simulink model "fukt_test"  (R2023b)
settings: Solver=FixedStepAuto  StartTime=0.0  StopTime=inf  FixedStep=0.5  MaxStep=1  MinStep=1  RelTol=1e-3
undefined symbols (not defined in the file or in its folder): BOOL, DINT, OTL, slplc
libraries: arduinolib x3
(part 5 of 6)

== system fukt_test/PLC Controller Suite/__Logic/Fukt logic/Program/__Logic/OTU1/RungInOverride/ForceRungInFalseRead/__CoreLabelRead ==
  DataRead : DataStoreRead  DataStoreName=x_PLCLabel__s4_3653__Force_RungIn_False  IndexOptions=Index vector (dialog)  Indices=1  OutputSizes=1
  Out1 : Outport  VectorParamsAs1DForOutWhenUnconnected=off
  wires:
  DataRead/1 -> Out1/1

== system fukt_test/PLC Controller Suite/__Logic/Fukt logic/Program/__Logic/OTU2/Instruction_Enable/Rung-condition-in is true/__CoreVarWrite ==
  u : Inport
  DataWrite : DataStoreWrite  DataStoreName=xxx_PLC_VAR_fukt_bool  IndexOptions=Index vector (dialog)  Indices=1  OutputSizes=1
  wires:
  u/1 -> DataWrite/1

== system fukt_test/PLC Controller Suite/__Logic/Fukt logic/Program/__Logic/OTU2/RungInOverride/ForceRungInFalseRead/__CoreLabelRead ==
  DataRead : DataStoreRead  DataStoreName=x_PLCLabel__s4_3653__Force_RungIn_False  IndexOptions=Index vector (dialog)  Indices=1  OutputSizes=1
  Out1 : Outport  VectorParamsAs1DForOutWhenUnconnected=off
  wires:
  DataRead/1 -> Out1/1

== system fukt_test/PLC Controller Suite/__Logic/Fukt logic/Program/__Logic/TON/Instruction_Enable/Initialize Function/VarWrite ==
  In1 : Inport
  __CoreVarWrite : Subsystem  Tag=CoreVarWriteBlock  DisableCoverage=on  TreatAsAtomicUnit=on  mask{PLCBlockType=CoreVarWrite}
      mask init:
      | slplc.callbacks.initCoreVariable(gcb, 'write');
      mask Help: web([docroot '/plccoder/ref/__corevarwrite' '.html']);
      mask DialogControl PLCBlockTitle Prompt: Core Variable Write
  wires:
  In1/1 -> __CoreVarWrite/1(u)

== system fukt_test/PLC Controller Suite/__Logic/Fukt logic/Program/__Logic/TON/Instruction_Enable/Initialize Function/VarWrite1 ==
  In1 : Inport
  __CoreVarWrite : Subsystem  Tag=CoreVarWriteBlock  DisableCoverage=on  TreatAsAtomicUnit=on  mask{PLCBlockType=CoreVarWrite}
      mask init:
      | slplc.callbacks.initCoreVariable(gcb, 'write');
      mask Help: web([docroot '/plccoder/ref/__corevarwrite' '.html']);
      mask DialogControl PLCBlockTitle Prompt: Core Variable Write
  wires:
  In1/1 -> __CoreVarWrite/1(u)

== system fukt_test/PLC Controller Suite/__Logic/Fukt logic/Program/__Logic/TON/Instruction_Enable/Initialize Function/VarWrite2 ==
  In1 : Inport
  __CoreVarWrite : Subsystem  Tag=CoreVarWriteBlock  DisableCoverage=on  TreatAsAtomicUnit=on  mask{PLCBlockType=CoreVarWrite}
      mask init:
      | slplc.callbacks.initCoreVariable(gcb, 'write');
      mask Help: web([docroot '/plccoder/ref/__corevarwrite' '.html']);
      mask DialogControl PLCBlockTitle Prompt: Core Variable Write
  wires:
  In1/1 -> __CoreVarWrite/1(u)

== system fukt_test/PLC Controller Suite/__Logic/Fukt logic/Program/__Logic/TON/Instruction_Enable/Initialize Function/VarWrite3 ==
  In1 : Inport
  __CoreVarWrite : Subsystem  Tag=CoreVarWriteBlock  DisableCoverage=on  TreatAsAtomicUnit=on  mask{PLCBlockType=CoreVarWrite}
      mask init:
      | slplc.callbacks.initCoreVariable(gcb, 'write');
      mask Help: web([docroot '/plccoder/ref/__corevarwrite' '.html']);
      mask DialogControl PLCBlockTitle Prompt: Core Variable Write
  wires:
  In1/1 -> __CoreVarWrite/1(u)

== system fukt_test/PLC Controller Suite/__Logic/Fukt logic/Program/__Logic/TON/RungInOverride/ForceRungInFalseRead/__CoreLabelRead ==
  DataRead : DataStoreRead  DataStoreName=x_PLCLabel__s4_3653__Force_RungIn_False  IndexOptions=Index vector (dialog)  Indices=1  OutputSizes=1
  Out1 : Outport  VectorParamsAs1DForOutWhenUnconnected=off
  wires:
  DataRead/1 -> Out1/1

== system fukt_test/PLC Controller Suite/__Logic/Fukt logic/Program/__Logic/XIC1/RungInOverride/ForceRungInFalseRead/__CoreLabelRead ==
  DataRead : DataStoreRead  DataStoreName=x_PLCLabel__s4_3653__Force_RungIn_False  IndexOptions=Index vector (dialog)  Indices=1  OutputSizes=1
  Out1 : Outport  VectorParamsAs1DForOutWhenUnconnected=off
  wires:
  DataRead/1 -> Out1/1

== system fukt_test/PLC Controller Suite/__Logic/Fukt logic/Program/__Logic/XIC2/RungInOverride/ForceRungInFalseRead/__CoreLabelRead ==
  DataRead : DataStoreRead  DataStoreName=x_PLCLabel__s4_3653__Force_RungIn_False  IndexOptions=Index vector (dialog)  Indices=1  OutputSizes=1
  Out1 : Outport  VectorParamsAs1DForOutWhenUnconnected=off
  wires:
  DataRead/1 -> Out1/1

== system fukt_test/PLC Controller Suite/__Logic/Fukt logic/Program/__Logic/XIC3/RungInOverride/ForceRungInFalseRead/__CoreLabelRead ==
  DataRead : DataStoreRead  DataStoreName=x_PLCLabel__s4_3653__Force_RungIn_False  IndexOptions=Index vector (dialog)  Indices=1  OutputSizes=1
  Out1 : Outport  VectorParamsAs1DForOutWhenUnconnected=off
  wires:
  DataRead/1 -> Out1/1

== system fukt_test/PLC Controller Suite/__Logic/Fukt sampling/Fuktmätare sampling/__Logic/MOV/RungInOverride/ForceRungInFalseRead/__CoreLabelRead ==
  DataRead : DataStoreRead  DataStoreName=x_PLCLabel__s4_3653__Force_RungIn_False  IndexOptions=Index vector (dialog)  Indices=1  OutputSizes=1
  Out1 : Outport  VectorParamsAs1DForOutWhenUnconnected=off
  wires:
  DataRead/1 -> Out1/1

== system fukt_test/PLC Controller Suite/__Logic/Fukt sampling/Fuktmätare sampling/__Logic/MOV/RungOutOverride/BlockEnableRead/__CoreLabelRead ==
  DataRead : DataStoreRead  DataStoreName=x_PLCLabel__s4_3653__Block_Enable  IndexOptions=Index vector (dialog)  Indices=1  OutputSizes=1
  Out1 : Outport  VectorParamsAs1DForOutWhenUnconnected=off
  wires:
  DataRead/1 -> Out1/1

== system fukt_test/PLC Controller Suite/__Logic/Fukt sampling/Fuktmätare sampling/__Logic/MOV/RungOutOverride/VariableWriteEnableWrite/__CoreLabelWrite ==
  In1 : Inport
  DataWrite : DataStoreWrite  DataStoreName=x_PLCLabel__s4_3653__Variable_Write_Enable  IndexOptions=Index vector (dialog)  Indices=1  OutputSizes=1
  wires:
  In1/1 -> DataWrite/1

== system fukt_test/PLC Controller Suite/__Logic/Fukt sampling/Fuktmätare sampling/__Logic/OTL/Instruction_Enable/Rung-condition-in is true/__CoreVarWrite ==
  u : Inport
  DataWrite : DataStoreWrite  DataStoreName=xxx_PLC_VAR_fukt_polling  IndexOptions=Index vector (dialog)  Indices=1  OutputSizes=1
  wires:
  u/1 -> DataWrite/1

== system fukt_test/PLC Controller Suite/__Logic/Fukt sampling/Fuktmätare sampling/__Logic/OTL/RungInOverride/ForceRungInFalseRead/__CoreLabelRead ==
  DataRead : DataStoreRead  DataStoreName=x_PLCLabel__s4_3653__Force_RungIn_False  IndexOptions=Index vector (dialog)  Indices=1  OutputSizes=1
  Out1 : Outport  VectorParamsAs1DForOutWhenUnconnected=off
  wires:
  DataRead/1 -> Out1/1

== system fukt_test/PLC Controller Suite/__Logic/Fukt sampling/Fuktmätare sampling/__Logic/OTL1/Instruction_Enable/Rung-condition-in is true/__CoreVarWrite ==
  u : Inport
  DataWrite : DataStoreWrite  DataStoreName=xxx_PLC_VAR_fukt_power  IndexOptions=Index vector (dialog)  Indices=1  OutputSizes=1
  wires:
  u/1 -> DataWrite/1

== system fukt_test/PLC Controller Suite/__Logic/Fukt sampling/Fuktmätare sampling/__Logic/OTL1/RungInOverride/ForceRungInFalseRead/__CoreLabelRead ==
  DataRead : DataStoreRead  DataStoreName=x_PLCLabel__s4_3653__Force_RungIn_False  IndexOptions=Index vector (dialog)  Indices=1  OutputSizes=1
  Out1 : Outport  VectorParamsAs1DForOutWhenUnconnected=off
  wires:
  DataRead/1 -> Out1/1

== system fukt_test/PLC Controller Suite/__Logic/Fukt sampling/Fuktmätare sampling/__Logic/OTU/Instruction_Enable/Rung-condition-in is true/__CoreVarWrite ==
  u : Inport
  DataWrite : DataStoreWrite  DataStoreName=xxx_PLC_VAR_fukt_power  IndexOptions=Index vector (dialog)  Indices=1  OutputSizes=1
  wires:
  u/1 -> DataWrite/1

== system fukt_test/PLC Controller Suite/__Logic/Fukt sampling/Fuktmätare sampling/__Logic/OTU/RungInOverride/ForceRungInFalseRead/__CoreLabelRead ==
  DataRead : DataStoreRead  DataStoreName=x_PLCLabel__s4_3653__Force_RungIn_False  IndexOptions=Index vector (dialog)  Indices=1  OutputSizes=1
  Out1 : Outport  VectorParamsAs1DForOutWhenUnconnected=off
  wires:
  DataRead/1 -> Out1/1

== system fukt_test/PLC Controller Suite/__Logic/Fukt sampling/Fuktmätare sampling/__Logic/RES/Instruction_Enable/Rung-condition-in is true/__CoreVarRead ==
  DataRead : DataStoreRead  DataStoreName=xxx_PLC_VAR_Fukt_periodicity  IndexOptions=Index vector (dialog)  Indices=1  OutputSizes=1
  y : Outport  VectorParamsAs1DForOutWhenUnconnected=off
  wires:
  DataRead/1 -> y/1

== system fukt_test/PLC Controller Suite/__Logic/Fukt sampling/Fuktmätare sampling/__Logic/RES/Instruction_Enable/Rung-condition-in is true/__CoreVarWrite ==
  u : Inport
  DataWrite : DataStoreWrite  DataStoreName=xxx_PLC_VAR_Fukt_periodicity  IndexOptions=Index vector (dialog)  Indices=1  OutputSizes=1
  wires:
  u/1 -> DataWrite/1

== system fukt_test/PLC Controller Suite/__Logic/Fukt sampling/Fuktmätare sampling/__Logic/RES/RungInOverride/ForceRungInFalseRead/__CoreLabelRead ==
  DataRead : DataStoreRead  DataStoreName=x_PLCLabel__s4_3653__Force_RungIn_False  IndexOptions=Index vector (dialog)  Indices=1  OutputSizes=1
  Out1 : Outport  VectorParamsAs1DForOutWhenUnconnected=off
  wires:
  DataRead/1 -> Out1/1

== system fukt_test/PLC Controller Suite/__Logic/Fukt sampling/Fuktmätare sampling/__Logic/TON/Instruction_Enable/Initialize Function/VarWrite ==
  In1 : Inport
  __CoreVarWrite : Subsystem  Tag=CoreVarWriteBlock  DisableCoverage=on  TreatAsAtomicUnit=on  mask{PLCBlockType=CoreVarWrite}
      mask init:
      | slplc.callbacks.initCoreVariable(gcb, 'write');
      mask Help: web([docroot '/plccoder/ref/__corevarwrite' '.html']);
      mask DialogControl PLCBlockTitle Prompt: Core Variable Write
  wires:
  In1/1 -> __CoreVarWrite/1(u)

== system fukt_test/PLC Controller Suite/__Logic/Fukt sampling/Fuktmätare sampling/__Logic/TON/Instruction_Enable/Initialize Function/VarWrite1 ==
  In1 : Inport
  __CoreVarWrite : Subsystem  Tag=CoreVarWriteBlock  DisableCoverage=on  TreatAsAtomicUnit=on  mask{PLCBlockType=CoreVarWrite}
      mask init:
      | slplc.callbacks.initCoreVariable(gcb, 'write');
      mask Help: web([docroot '/plccoder/ref/__corevarwrite' '.html']);
      mask DialogControl PLCBlockTitle Prompt: Core Variable Write
  wires:
  In1/1 -> __CoreVarWrite/1(u)

== system fukt_test/PLC Controller Suite/__Logic/Fukt sampling/Fuktmätare sampling/__Logic/TON/Instruction_Enable/Initialize Function/VarWrite2 ==
  In1 : Inport
  __CoreVarWrite : Subsystem  Tag=CoreVarWriteBlock  DisableCoverage=on  TreatAsAtomicUnit=on  mask{PLCBlockType=CoreVarWrite}
      mask init:
      | slplc.callbacks.initCoreVariable(gcb, 'write');
      mask Help: web([docroot '/plccoder/ref/__corevarwrite' '.html']);
      mask DialogControl PLCBlockTitle Prompt: Core Variable Write
  wires:
  In1/1 -> __CoreVarWrite/1(u)

== system fukt_test/PLC Controller Suite/__Logic/Fukt sampling/Fuktmätare sampling/__Logic/TON/Instruction_Enable/Initialize Function/VarWrite3 ==
  In1 : Inport
  __CoreVarWrite : Subsystem  Tag=CoreVarWriteBlock  DisableCoverage=on  TreatAsAtomicUnit=on  mask{PLCBlockType=CoreVarWrite}
      mask init:
      | slplc.callbacks.initCoreVariable(gcb, 'write');
      mask Help: web([docroot '/plccoder/ref/__corevarwrite' '.html']);
      mask DialogControl PLCBlockTitle Prompt: Core Variable Write
  wires:
  In1/1 -> __CoreVarWrite/1(u)

== system fukt_test/PLC Controller Suite/__Logic/Fukt sampling/Fuktmätare sampling/__Logic/TON/RungInOverride/ForceRungInFalseRead/__CoreLabelRead ==
  DataRead : DataStoreRead  DataStoreName=x_PLCLabel__s4_3653__Force_RungIn_False  IndexOptions=Index vector (dialog)  Indices=1  OutputSizes=1
  Out1 : Outport  VectorParamsAs1DForOutWhenUnconnected=off
  wires:
  DataRead/1 -> Out1/1

== system fukt_test/PLC Controller Suite/__Logic/Fukt sampling/Fuktmätare sampling/__Logic/TON1/Instruction_Enable/Initialize Function/VarWrite ==
  In1 : Inport
  __CoreVarWrite : Subsystem  Tag=CoreVarWriteBlock  DisableCoverage=on  TreatAsAtomicUnit=on  mask{PLCBlockType=CoreVarWrite}
      mask init:
      | slplc.callbacks.initCoreVariable(gcb, 'write');
      mask Help: web([docroot '/plccoder/ref/__corevarwrite' '.html']);
      mask DialogControl PLCBlockTitle Prompt: Core Variable Write
  wires:
  In1/1 -> __CoreVarWrite/1(u)

== system fukt_test/PLC Controller Suite/__Logic/Fukt sampling/Fuktmätare sampling/__Logic/TON1/Instruction_Enable/Initialize Function/VarWrite1 ==
  In1 : Inport
  __CoreVarWrite : Subsystem  Tag=CoreVarWriteBlock  DisableCoverage=on  TreatAsAtomicUnit=on  mask{PLCBlockType=CoreVarWrite}
      mask init:
      | slplc.callbacks.initCoreVariable(gcb, 'write');
      mask Help: web([docroot '/plccoder/ref/__corevarwrite' '.html']);
      mask DialogControl PLCBlockTitle Prompt: Core Variable Write
  wires:
  In1/1 -> __CoreVarWrite/1(u)

== system fukt_test/PLC Controller Suite/__Logic/Fukt sampling/Fuktmätare sampling/__Logic/TON1/Instruction_Enable/Initialize Function/VarWrite2 ==
  In1 : Inport
  __CoreVarWrite : Subsystem  Tag=CoreVarWriteBlock  DisableCoverage=on  TreatAsAtomicUnit=on  mask{PLCBlockType=CoreVarWrite}
      mask init:
      | slplc.callbacks.initCoreVariable(gcb, 'write');
      mask Help: web([docroot '/plccoder/ref/__corevarwrite' '.html']);
      mask DialogControl PLCBlockTitle Prompt: Core Variable Write
  wires:
  In1/1 -> __CoreVarWrite/1(u)

== system fukt_test/PLC Controller Suite/__Logic/Fukt sampling/Fuktmätare sampling/__Logic/TON1/Instruction_Enable/Initialize Function/VarWrite3 ==
  In1 : Inport
  __CoreVarWrite : Subsystem  Tag=CoreVarWriteBlock  DisableCoverage=on  TreatAsAtomicUnit=on  mask{PLCBlockType=CoreVarWrite}
      mask init:
      | slplc.callbacks.initCoreVariable(gcb, 'write');
      mask Help: web([docroot '/plccoder/ref/__corevarwrite' '.html']);
      mask DialogControl PLCBlockTitle Prompt: Core Variable Write
  wires:
  In1/1 -> __CoreVarWrite/1(u)

== system fukt_test/PLC Controller Suite/__Logic/Fukt sampling/Fuktmätare sampling/__Logic/TON1/RungInOverride/ForceRungInFalseRead/__CoreLabelRead ==
  DataRead : DataStoreRead  DataStoreName=x_PLCLabel__s4_3653__Force_RungIn_False  IndexOptions=Index vector (dialog)  Indices=1  OutputSizes=1
  Out1 : Outport  VectorParamsAs1DForOutWhenUnconnected=off
  wires:
  DataRead/1 -> Out1/1

== system fukt_test/PLC Controller Suite/__Logic/Fukt sampling/Fuktmätare sampling/__Logic/XIC1/RungInOverride/ForceRungInFalseRead/__CoreLabelRead ==
  DataRead : DataStoreRead  DataStoreName=x_PLCLabel__s4_3653__Force_RungIn_False  IndexOptions=Index vector (dialog)  Indices=1  OutputSizes=1
  Out1 : Outport  VectorParamsAs1DForOutWhenUnconnected=off
  wires:
  DataRead/1 -> Out1/1

== system fukt_test/PLC Controller Suite/__Logic/Fukt sampling/Fuktmätare sampling/__Logic/XIC2/RungInOverride/ForceRungInFalseRead/__CoreLabelRead ==
  DataRead : DataStoreRead  DataStoreName=x_PLCLabel__s4_3653__Force_RungIn_False  IndexOptions=Index vector (dialog)  Indices=1  OutputSizes=1
  Out1 : Outport  VectorParamsAs1DForOutWhenUnconnected=off
  wires:
  DataRead/1 -> Out1/1

== system fukt_test/PLC Controller Suite/__Logic/Fukt logic/Program/__Logic/TON/Instruction_Enable/Initialize Function/VarWrite/__CoreVarWrite ==
  u : Inport
  DataWrite : DataStoreWrite  DataStoreName=xxx_PLC_VAR_orange_led_timer_1  DataStoreElements=xxx_PLC_VAR_orange_led_timer_1.ACC  IndexOptions=Index vector (dialog)  Indices=1  OutputSizes=1
  wires:
  u/1 -> DataWrite/1

== system fukt_test/PLC Controller Suite/__Logic/Fukt logic/Program/__Logic/TON/Instruction_Enable/Initialize Function/VarWrite1/__CoreVarWrite ==
  u : Inport
  DataWrite : DataStoreWrite  DataStoreName=xxx_PLC_VAR_orange_led_timer_1  DataStoreElements=xxx_PLC_VAR_orange_led_timer_1.EN  IndexOptions=Index vector (dialog)  Indices=1  OutputSizes=1
  wires:
  u/1 -> DataWrite/1

== system fukt_test/PLC Controller Suite/__Logic/Fukt logic/Program/__Logic/TON/Instruction_Enable/Initialize Function/VarWrite2/__CoreVarWrite ==
  u : Inport
  DataWrite : DataStoreWrite  DataStoreName=xxx_PLC_VAR_orange_led_timer_1  DataStoreElements=xxx_PLC_VAR_orange_led_timer_1.TT  IndexOptions=Index vector (dialog)  Indices=1  OutputSizes=1
  wires:
  u/1 -> DataWrite/1

== system fukt_test/PLC Controller Suite/__Logic/Fukt logic/Program/__Logic/TON/Instruction_Enable/Initialize Function/VarWrite3/__CoreVarWrite ==
  u : Inport
  DataWrite : DataStoreWrite  DataStoreName=xxx_PLC_VAR_orange_led_timer_1  DataStoreElements=xxx_PLC_VAR_orange_led_timer_1.DN  IndexOptions=Index vector (dialog)  Indices=1  OutputSizes=1
  wires:
  u/1 -> DataWrite/1

== system fukt_test/PLC Controller Suite/__Logic/Fukt sampling/Fuktmätare sampling/__Logic/TON/Instruction_Enable/Initialize Function/VarWrite/__CoreVarWrite ==
  u : Inport
  DataWrite : DataStoreWrite  DataStoreName=xxx_PLC_VAR_Fukt_periodicity  DataStoreElements=xxx_PLC_VAR_Fukt_periodicity.ACC  IndexOptions=Index vector (dialog)  Indices=1  OutputSizes=1
  wires:
  u/1 -> DataWrite/1

== system fukt_test/PLC Controller Suite/__Logic/Fukt sampling/Fuktmätare sampling/__Logic/TON/Instruction_Enable/Initialize Function/VarWrite1/__CoreVarWrite ==
  u : Inport
  DataWrite : DataStoreWrite  DataStoreName=xxx_PLC_VAR_Fukt_periodicity  DataStoreElements=xxx_PLC_VAR_Fukt_periodicity.EN  IndexOptions=Index vector (dialog)  Indices=1  OutputSizes=1
  wires:
  u/1 -> DataWrite/1

== system fukt_test/PLC Controller Suite/__Logic/Fukt sampling/Fuktmätare sampling/__Logic/TON/Instruction_Enable/Initialize Function/VarWrite2/__CoreVarWrite ==
  u : Inport
  DataWrite : DataStoreWrite  DataStoreName=xxx_PLC_VAR_Fukt_periodicity  DataStoreElements=xxx_PLC_VAR_Fukt_periodicity.TT  IndexOptions=Index vector (dialog)  Indices=1  OutputSizes=1
  wires:
  u/1 -> DataWrite/1

== system fukt_test/PLC Controller Suite/__Logic/Fukt sampling/Fuktmätare sampling/__Logic/TON/Instruction_Enable/Initialize Function/VarWrite3/__CoreVarWrite ==
  u : Inport
  DataWrite : DataStoreWrite  DataStoreName=xxx_PLC_VAR_Fukt_periodicity  DataStoreElements=xxx_PLC_VAR_Fukt_periodicity.DN  IndexOptions=Index vector (dialog)  Indices=1  OutputSizes=1
  wires:
  u/1 -> DataWrite/1

== system fukt_test/PLC Controller Suite/__Logic/Fukt sampling/Fuktmätare sampling/__Logic/TON1/Instruction_Enable/Initialize Function/VarWrite/__CoreVarWrite ==
  u : Inport
  DataWrite : DataStoreWrite  DataStoreName=xxx_PLC_VAR_d13_wait  DataStoreElements=xxx_PLC_VAR_d13_wait.ACC  IndexOptions=Index vector (dialog)  Indices=1  OutputSizes=1
  wires:
  u/1 -> DataWrite/1

== system fukt_test/PLC Controller Suite/__Logic/Fukt sampling/Fuktmätare sampling/__Logic/TON1/Instruction_Enable/Initialize Function/VarWrite1/__CoreVarWrite ==
  u : Inport
  DataWrite : DataStoreWrite  DataStoreName=xxx_PLC_VAR_d13_wait  DataStoreElements=xxx_PLC_VAR_d13_wait.EN  IndexOptions=Index vector (dialog)  Indices=1  OutputSizes=1
  wires:
  u/1 -> DataWrite/1

== system fukt_test/PLC Controller Suite/__Logic/Fukt sampling/Fuktmätare sampling/__Logic/TON1/Instruction_Enable/Initialize Function/VarWrite2/__CoreVarWrite ==
  u : Inport
  DataWrite : DataStoreWrite  DataStoreName=xxx_PLC_VAR_d13_wait  DataStoreElements=xxx_PLC_VAR_d13_wait.TT  IndexOptions=Index vector (dialog)  Indices=1  OutputSizes=1
  wires:
  u/1 -> DataWrite/1

== system fukt_test/PLC Controller Suite/__Logic/Fukt sampling/Fuktmätare sampling/__Logic/TON1/Instruction_Enable/Initialize Function/VarWrite3/__CoreVarWrite ==
  u : Inport
  DataWrite : DataStoreWrite  DataStoreName=xxx_PLC_VAR_d13_wait  DataStoreElements=xxx_PLC_VAR_d13_wait.DN  IndexOptions=Index vector (dialog)  Indices=1  OutputSizes=1
  wires:
  u/1 -> DataWrite/1

== matlab function fukt_test/PLC Controller Suite/__Logic/Fukt sampling/Fuktmätare sampling/__Logic/Power Rail Start/__Format ==
  data: RungOut input
function setBlockFormat(RungOut)
% set parent block colors
coder.extrinsic('slplc.utils.setBlockAppearance');
persistent isInit lastRungOut lastAnimation lastRungOutShow;

if isempty(isInit)
    isInit = true;
else
    isInit = false;
end

if isempty(lastRungOut)
    lastRungOut = RungOut;
end

if isempty(lastAnimation)
    lastAnimation = false;
end

if isempty(lastRungOutShow)
    lastRungOutShow = false;
end

[animation, dataShow] = slplc.utils.setBlockAppearance('set', '', {'black', 'black'}, {}, ...
    '', {'ForegroundColor', 'BackgroundColor'}, ...
    isInit,  ...
    true,  true, ...
    RungOut,   lastRungOut, ...
    RungOut,   lastRungOut, ...
    [],    [], ...
    lastAnimation, lastRungOutShow);

lastRungOut         = RungOut;
lastAnimation       = animation;
lastRungOutShow     = dataShow;
end

== matlab function fukt_test/PLC Controller Suite/__Logic/Fukt logic/Program/__Logic/TON/Instruction_Enable/__Logic ==
  data: EN output; TT output; RungIn input; PRE input; EN input; DN input; DN output; ACC output; ACC input; currentTime input; lastTime input
function [EN, TT, DN, ACC]  = TON(RungIn, PRE, EN, DN, ACC, currentTime, lastTime)
% TON algorithm

if RungIn
    % Rung-condition-in is True
    if PRE < 0 || ACC < 0
        error('slplc:TONError', '.PRE or .ACC cannot be negtive values');
    end
    TT = true;
    if ~DN
        if EN
            deltaT = currentTime - lastTime;
            ACC = ACC + cast(deltaT, class(ACC));
            if ACC == intmax(class(ACC)) || ACC >= PRE
                TT = false;
                DN = true;
            end
        end
    else
        TT = false;
    end
    EN = true;
    % True end
else
    % Rung-condition-in is False
    EN    = false;
    TT    = false;
    DN    = false;
    ACC   = cast(0, class(ACC));
    % False end
end

end

== matlab function fukt_test/PLC Controller Suite/__Logic/Fukt sampling/Fuktmätare sampling/__Logic/TON/Instruction_Enable/__Logic ==
  data: EN output; TT output; RungIn input; PRE input; EN input; DN input; DN output; ACC output; ACC input; currentTime input; lastTime input
function [EN, TT, DN, ACC]  = TON(RungIn, PRE, EN, DN, ACC, currentTime, lastTime)
% TON algorithm

if RungIn
    % Rung-condition-in is True
    if PRE < 0 || ACC < 0
        error('slplc:TONError', '.PRE or .ACC cannot be negtive values');
    end
    TT = true;
    if ~DN
        if EN
            deltaT = currentTime - lastTime;
            ACC = ACC + cast(deltaT, class(ACC));
            if ACC == intmax(class(ACC)) || ACC >= PRE
                TT = false;
                DN = true;
            end
        end
    else
        TT = false;
    end
    EN = true;
    % True end
else
    % Rung-condition-in is False
    EN    = false;
    TT    = false;
    DN    = false;
    ACC   = cast(0, class(ACC));
    % False end
end

end

== matlab function fukt_test/PLC Controller Suite/__Logic/Fukt sampling/Fuktmätare sampling/__Logic/TON/__Format ==
  data: BlockEnable input; RungIn input; RungOut input; data input
function setBlockFormat(BlockEnable, RungIn, RungOut, data)
% set parent block colors
coder.extrinsic('slplc.utils.setBlockAppearance');
persistent lastBlockEnable lastRungIn lastRungOut lastData isInit lastAnimation lastDataShow;
if isempty(lastBlockEnable)
    lastBlockEnable = true;
end
if isempty(lastRungIn)
    lastRungIn = false;
end
if isempty(lastRungOut)
    lastRungOut = false;
end
if isempty(lastData)
    lastData = data;
end
if isempty(isInit)
    isInit = true;
else
    isInit = false;
end
if isempty(lastAnimation)
    lastAnimation = false;
end
if isempty(lastDataShow)
    lastDataShow = false;
end

[animation, dataShow] = slplc.utils.setBlockAppearance('set', '%<PLCBlockType>: %<PLCOperandTag>', {}, {}, ...
    ' = ', {'ForegroundColor'}, ...
    isInit,  ...
    BlockEnable, lastBlockEnable, ...
    RungIn,  lastRungIn, ...
    RungOut, lastRungOut, ...
    data, lastData, ...
    lastAnimation, lastDataShow);

lastBlockEnable = BlockEnable;
lastRungIn      = RungIn;
lastRungOut     = RungOut;
lastData        = data;
lastAnimation   = animation;
lastDataShow    = dataShow;
end

== matlab function fukt_test/PLC Controller Suite/__Logic/Fukt sampling/Fuktmätare sampling/__Logic/Variable Read/__Format ==
  data: data input
function setBlockFormat(data)
% set parent block colors
coder.extrinsic('slplc.utils.setBlockAppearance');
persistent isInit lastData  lastAnimation lastDataShow;

if isempty(isInit)
    isInit = true;
else
    isInit = false;
end

if isempty(lastData)
    lastData = data;
end

if isempty(lastAnimation)
    lastAnimation = false;
end

if isempty(lastDataShow)
    lastDataShow = false;
end

[animation, dataShow] = slplc.utils.setBlockAppearance('set', '', {}, {}, ...
    '%<PLCOperandTag> = ', {}, ...
    isInit,  ...
    true,  true, ...
    false, false, ...
    false, false, ...
    data,  lastData, ...
    lastAnimation, lastDataShow);

lastData        = data;
lastAnimation   = animation;
lastDataShow    = dataShow;
end

== matlab function fukt_test/PLC Controller Suite/__Logic/Fukt logic/Program/__Logic/TON/__Format ==
  data: BlockEnable input; RungIn input; RungOut input; data input
function setBlockFormat(BlockEnable, RungIn, RungOut, data)
% set parent block colors
coder.extrinsic('slplc.utils.setBlockAppearance');
persistent lastBlockEnable lastRungIn lastRungOut lastData isInit lastAnimation lastDataShow;
if isempty(lastBlockEnable)
    lastBlockEnable = true;
end
if isempty(lastRungIn)
    lastRungIn = false;
end
if isempty(lastRungOut)
    lastRungOut = false;
end
if isempty(lastData)
    lastData = data;
end
if isempty(isInit)
    isInit = true;
else
    isInit = false;
end
if isempty(lastAnimation)
    lastAnimation = false;
end
if isempty(lastDataShow)
    lastDataShow = false;
end

[animation, dataShow] = slplc.utils.setBlockAppearance('set', '%<PLCBlockType>: %<PLCOperandTag>', {}, {}, ...
    ' = ', {'ForegroundColor'}, ...
    isInit,  ...
    BlockEnable, lastBlockEnable, ...
    RungIn,  lastRungIn, ...
    RungOut, lastRungOut, ...
    data, lastData, ...
    lastAnimation, lastDataShow);

lastBlockEnable = BlockEnable;
lastRungIn      = RungIn;
lastRungOut     = RungOut;
lastData        = data;
lastAnimation   = animation;
lastDataShow    = dataShow;
end

== matlab function fukt_test/PLC Controller Suite/__Logic/Fukt logic/Program/__Logic/OTU/__Format ==
  data: BlockEnable input; RungIn input; RungOut input; data input
function setBlockFormat(BlockEnable, RungIn, RungOut, data)

if data~=0 && data~=1
    error('slplc:inivalidBooleanValue', 'Invalid boolean value %d', data);
end
data = logical(data);

% set parent block colors
coder.extrinsic('slplc.utils.setBlockAppearance');
persistent lastBlockEnable lastRungIn lastRungOut lastData isInit lastAnimation lastDataShow;
if isempty(lastBlockEnable)
    lastBlockEnable = true;
end
if isempty(lastRungIn)
    lastRungIn = false;
end
if isempty(lastRungOut)
    lastRungOut = false;
end
if isempty(lastData)
    lastData = data;
end
if isempty(isInit)
    isInit = true;
else
    isInit = false;
end
if isempty(lastAnimation)
    lastAnimation = false;
end
if isempty(lastDataShow)
    lastDataShow = false;
end

[animation, dataShow] = slplc.utils.setBlockAppearance('set', '%<PLCOperandTag>', {}, {}, ...
    ' = ', {'ForegroundColor'}, ...
    isInit,  ...
    BlockEnable, lastBlockEnable, ...
    RungIn,  lastRungIn, ...
    RungOut, lastRungOut, ...
    data, lastData, ...
    lastAnimation, lastDataShow);

lastBlockEnable = BlockEnable;
lastRungIn      = RungIn;
lastRungOut     = RungOut;
lastData        = data;
lastAnimation   = animation;
lastDataShow    = dataShow;
end

== matlab function fukt_test/PLC Controller Suite/__Logic/Fukt logic/Program/__Logic/OTU1/__Format ==
  data: BlockEnable input; RungIn input; RungOut input; data input
function setBlockFormat(BlockEnable, RungIn, RungOut, data)

if data~=0 && data~=1
    error('slplc:inivalidBooleanValue', 'Invalid boolean value %d', data);
end
data = logical(data);

% set parent block colors
coder.extrinsic('slplc.utils.setBlockAppearance');
persistent lastBlockEnable lastRungIn lastRungOut lastData isInit lastAnimation lastDataShow;
if isempty(lastBlockEnable)
    lastBlockEnable = true;
end
if isempty(lastRungIn)
    lastRungIn = false;
end
if isempty(lastRungOut)
    lastRungOut = false;
end
if isempty(lastData)
    lastData = data;
end
if isempty(isInit)
    isInit = true;
else
    isInit = false;
end
if isempty(lastAnimation)
    lastAnimation = false;
end
if isempty(lastDataShow)
    lastDataShow = false;
end

[animation, dataShow] = slplc.utils.setBlockAppearance('set', '%<PLCOperandTag>', {}, {}, ...
    ' = ', {'ForegroundColor'}, ...
    isInit,  ...
    BlockEnable, lastBlockEnable, ...
    RungIn,  lastRungIn, ...
    RungOut, lastRungOut, ...
    data, lastData, ...
    lastAnimation, lastDataShow);

lastBlockEnable = BlockEnable;
lastRungIn      = RungIn;
lastRungOut     = RungOut;
lastData        = data;
lastAnimation   = animation;
lastDataShow    = dataShow;
end

== matlab function fukt_test/PLC Controller Suite/__Logic/Fukt sampling/Fuktmätare sampling/__Logic/Variable Write/__Format ==
  data: data input
function setBlockFormat(data)
% set parent block colors
coder.extrinsic('slplc.utils.setBlockAppearance');
persistent isInit lastData  lastAnimation lastDataShow;

if isempty(isInit)
    isInit = true;
else
    isInit = false;
end

if isempty(lastData)
    lastData = data;
end

if isempty(lastAnimation)
    lastAnimation = false;
end

if isempty(lastDataShow)
    lastDataShow = false;
end

[animation, dataShow] = slplc.utils.setBlockAppearance('set', '', {}, {}, ...
    '%<PLCOperandTag> = ', {}, ...
    isInit,  ...
    true,  true, ...
    false, false, ...
    false, false, ...
    data,  lastData, ...
    lastAnimation, lastDataShow);

lastData        = data;
lastAnimation   = animation;
lastDataShow    = dataShow;
end

== matlab function fukt_test/PLC Controller Suite/__Logic/Fukt sampling/Fuktmätare sampling/__Logic/OTL/__Format ==
  data: BlockEnable input; RungIn input; RungOut input; data input
function setBlockFormat(BlockEnable, RungIn, RungOut, data)

if data~=0 && data~=1
    error('slplc:inivalidBooleanValue', 'Invalid boolean value %d', data);
end
data = logical(data);

% set parent block colors
coder.extrinsic('slplc.utils.setBlockAppearance');
persistent lastBlockEnable lastRungIn lastRungOut lastData isInit lastAnimation lastDataShow;
if isempty(lastBlockEnable)
    lastBlockEnable = true;
end
if isempty(lastRungIn)
    lastRungIn = false;
end
if isempty(lastRungOut)
    lastRungOut = false;
end
if isempty(lastData)
    lastData = data;
end
if isempty(isInit)
    isInit = true;
else
    isInit = false;
end
if isempty(lastAnimation)
    lastAnimation = false;
end
if isempty(lastDataShow)
    lastDataShow = false;
end

[animation, dataShow] = slplc.utils.setBlockAppearance('set', '%<PLCOperandTag>', {}, {}, ...
    ' = ', {'ForegroundColor'}, ...
    isInit,  ...
    BlockEnable, lastBlockEnable, ...
    RungIn,  lastRungIn, ...
    RungOut, lastRungOut, ...
    data, lastData, ...
    lastAnimation, lastDataShow);

lastBlockEnable = BlockEnable;
lastRungIn      = RungIn;
lastRungOut     = RungOut;
lastData        = data;
lastAnimation   = animation;
lastDataShow    = dataShow;
end

== matlab function fukt_test/PLC Controller Suite/__Logic/Fukt logic/Program/__Logic/XIC3/__Format ==
  data: BlockEnable input; RungIn input; RungOut input; data input
function setBlockFormat(BlockEnable, RungIn, RungOut, data)

if data~=0 && data~=1
    error('slplc:inivalidBooleanValue', 'Invalid boolean value %d', data);
end
data = logical(data);

% set parent block colors
coder.extrinsic('slplc.utils.setBlockAppearance');
persistent lastBlockEnable lastRungIn lastRungOut lastData isInit lastAnimation lastDataShow;
if isempty(lastBlockEnable)
    lastBlockEnable = true;
end
if isempty(lastRungIn)
    lastRungIn = false;
end
if isempty(lastRungOut)
    lastRungOut = false;
end
if isempty(lastData)
    lastData = data;
end
if isempty(isInit)
    isInit = true;
else
    isInit = false;
end
if isempty(lastAnimation)
    lastAnimation = false;
end
if isempty(lastDataShow)
    lastDataShow = false;
end

[animation, dataShow] = slplc.utils.setBlockAppearance('set', '%<PLCOperandTag>', {}, {}, ...
    ' = ', {'ForegroundColor'}, ...
    isInit,  ...
    BlockEnable, lastBlockEnable, ...
    RungIn,  lastRungIn, ...
    RungOut, lastRungOut, ...
    data, lastData, ...
    lastAnimation, lastDataShow);

lastBlockEnable = BlockEnable;
lastRungIn      = RungIn;
lastRungOut     = RungOut;
lastData        = data;
lastAnimation   = animation;
lastDataShow    = dataShow;
end

== matlab function fukt_test/PLC Controller Suite/__Logic/Fukt logic/Program/__Logic/XIC1/__Format ==
  data: BlockEnable input; RungIn input; RungOut input; data input
function setBlockFormat(BlockEnable, RungIn, RungOut, data)

if data~=0 && data~=1
    error('slplc:inivalidBooleanValue', 'Invalid boolean value %d', data);
end
data = logical(data);

% set parent block colors
coder.extrinsic('slplc.utils.setBlockAppearance');
persistent lastBlockEnable lastRungIn lastRungOut lastData isInit lastAnimation lastDataShow;
if isempty(lastBlockEnable)
    lastBlockEnable = true;
end
if isempty(lastRungIn)
    lastRungIn = false;
end
if isempty(lastRungOut)
    lastRungOut = false;
end
if isempty(lastData)
    lastData = data;
end
if isempty(isInit)
    isInit = true;
else
    isInit = false;
end
if isempty(lastAnimation)
    lastAnimation = false;
end
if isempty(lastDataShow)
    lastDataShow = false;
end

[animation, dataShow] = slplc.utils.setBlockAppearance('set', '%<PLCOperandTag>', {}, {}, ...
    ' = ', {'ForegroundColor'}, ...
    isInit,  ...
    BlockEnable, lastBlockEnable, ...
    RungIn,  lastRungIn, ...
    RungOut, lastRungOut, ...
    data, lastData, ...
    lastAnimation, lastDataShow);

lastBlockEnable = BlockEnable;
lastRungIn      = RungIn;
lastRungOut     = RungOut;
lastData        = data;
lastAnimation   = animation;
lastDataShow    = dataShow;
end

== matlab function fukt_test/PLC Controller Suite/__Logic/Fukt logic/Program/__Logic/XIC2/__Format ==
  data: BlockEnable input; RungIn input; RungOut input; data input
function setBlockFormat(BlockEnable, RungIn, RungOut, data)

if data~=0 && data~=1
    error('slplc:inivalidBooleanValue', 'Invalid boolean value %d', data);
end
data = logical(data);

% set parent block colors
coder.extrinsic('slplc.utils.setBlockAppearance');
persistent lastBlockEnable lastRungIn lastRungOut lastData isInit lastAnimation lastDataShow;
if isempty(lastBlockEnable)
    lastBlockEnable = true;
end
if isempty(lastRungIn)
    lastRungIn = false;
end
if isempty(lastRungOut)
    lastRungOut = false;
end
if isempty(lastData)
    lastData = data;
end
if isempty(isInit)
    isInit = true;
else
    isInit = false;
end
if isempty(lastAnimation)
    lastAnimation = false;
end
if isempty(lastDataShow)
    lastDataShow = false;
end

[animation, dataShow] = slplc.utils.setBlockAppearance('set', '%<PLCOperandTag>', {}, {}, ...
    ' = ', {'ForegroundColor'}, ...
    isInit,  ...
    BlockEnable, lastBlockEnable, ...
    RungIn,  lastRungIn, ...
    RungOut, lastRungOut, ...
    data, lastData, ...
    lastAnimation, lastDataShow);

lastBlockEnable = BlockEnable;
lastRungIn      = RungIn;
lastRungOut     = RungOut;
lastData        = data;
lastAnimation   = animation;
lastDataShow    = dataShow;
end

== matlab function fukt_test/PLC Controller Suite/__Logic/Fukt logic/Program/__Logic/GEQ/__Format ==
  data: BlockEnable input; RungIn input; RungOut input
function setBlockFormat(BlockEnable, RungIn, RungOut)
% set parent block colors
coder.extrinsic('slplc.utils.setBlockAppearance');
persistent lastBlockEnable lastRungIn lastRungOut isInit lastAnimation lastDataShow;
if isempty(lastBlockEnable)
    lastBlockEnable = true;
end
if isempty(lastRungIn)
    lastRungIn = false;
end
if isempty(lastRungOut)
    lastRungOut = false;
end

if isempty(isInit)
    isInit = true;
else
    isInit = false;
end
if isempty(lastAnimation)
    lastAnimation = false;
end
if isempty(lastDataShow)
    lastDataShow = false;
end

[animation, dataShow] = slplc.utils.setBlockAppearance('set', '', {}, {}, ...
    ' = ',  {'ForegroundColor'}, ...
    isInit,  ...
    BlockEnable, lastBlockEnable, ...
    RungIn,  lastRungIn, ...
    RungOut, lastRungOut, ...
    [],    [], ...
    lastAnimation, lastDataShow);

lastBlockEnable = BlockEnable;
lastRungIn      = RungIn;
lastRungOut     = RungOut;
lastAnimation   = animation;
lastDataShow    = dataShow;
end

== matlab function fukt_test/PLC Controller Suite/__Logic/Fukt logic/Program/__Logic/Variable Read/__Format ==
  data: data input
function setBlockFormat(data)
% set parent block colors
coder.extrinsic('slplc.utils.setBlockAppearance');
persistent isInit lastData  lastAnimation lastDataShow;

if isempty(isInit)
    isInit = true;
else
    isInit = false;
end

if isempty(lastData)
    lastData = data;
end

if isempty(lastAnimation)
    lastAnimation = false;
end

if isempty(lastDataShow)
    lastDataShow = false;
end

[animation, dataShow] = slplc.utils.setBlockAppearance('set', '', {}, {}, ...
    '%<PLCOperandTag> = ', {}, ...
    isInit,  ...
    true,  true, ...
    false, false, ...
    false, false, ...
    data,  lastData, ...
    lastAnimation, lastDataShow);

lastData        = data;
lastAnimation   = animation;
lastDataShow    = dataShow;
end

== matlab function fukt_test/PLC Controller Suite/__Logic/Fukt logic/Program/__Logic/Variable Read1/__Format ==
  data: data input
function setBlockFormat(data)
% set parent block colors
coder.extrinsic('slplc.utils.setBlockAppearance');
persistent isInit lastData  lastAnimation lastDataShow;

if isempty(isInit)
    isInit = true;
else
    isInit = false;
end

if isempty(lastData)
    lastData = data;
end

if isempty(lastAnimation)
    lastAnimation = false;
end

if isempty(lastDataShow)
    lastDataShow = false;
end

[animation, dataShow] = slplc.utils.setBlockAppearance('set', '', {}, {}, ...
    '%<PLCOperandTag> = ', {}, ...
    isInit,  ...
    true,  true, ...
    false, false, ...
    false, false, ...
    data,  lastData, ...
    lastAnimation, lastDataShow);

lastData        = data;
lastAnimation   = animation;
lastDataShow    = dataShow;
end

== matlab function fukt_test/PLC Controller Suite/__Logic/Fukt sampling/Fuktmätare sampling/__Logic/OTU/__Format ==
  data: BlockEnable input; RungIn input; RungOut input; data input
function setBlockFormat(BlockEnable, RungIn, RungOut, data)

if data~=0 && data~=1
    error('slplc:inivalidBooleanValue', 'Invalid boolean value %d', data);
end
data = logical(data);

% set parent block colors
coder.extrinsic('slplc.utils.setBlockAppearance');
persistent lastBlockEnable lastRungIn lastRungOut lastData isInit lastAnimation lastDataShow;
if isempty(lastBlockEnable)
    lastBlockEnable = true;
end
if isempty(lastRungIn)
    lastRungIn = false;
end
if isempty(lastRungOut)
    lastRungOut = false;
end
if isempty(lastData)
    lastData = data;
end
if isempty(isInit)
    isInit = true;
else
    isInit = false;
end
if isempty(lastAnimation)
    lastAnimation = false;
end
if isempty(lastDataShow)
    lastDataShow = false;
end

[animation, dataShow] = slplc.utils.setBlockAppearance('set', '%<PLCOperandTag>', {}, {}, ...
    ' = ', {'ForegroundColor'}, ...
    isInit,  ...
    BlockEnable, lastBlockEnable, ...
    RungIn,  lastRungIn, ...
    RungOut, lastRungOut, ...
    data, lastData, ...
    lastAnimation, lastDataShow);

lastBlockEnable = BlockEnable;
lastRungIn      = RungIn;
lastRungOut     = RungOut;
lastData        = data;
lastAnimation   = animation;
lastDataShow    = dataShow;
end

== matlab function fukt_test/PLC Controller Suite/__Logic/Fukt sampling/Fuktmätare sampling/__Logic/OTL1/__Format ==
  data: BlockEnable input; RungIn input; RungOut input; data input
function setBlockFormat(BlockEnable, RungIn, RungOut, data)

if data~=0 && data~=1
    error('slplc:inivalidBooleanValue', 'Invalid boolean value %d', data);
end
data = logical(data);

% set parent block colors
coder.extrinsic('slplc.utils.setBlockAppearance');
persistent lastBlockEnable lastRungIn lastRungOut lastData isInit lastAnimation lastDataShow;
if isempty(lastBlockEnable)
    lastBlockEnable = true;
end
if isempty(lastRungIn)
    lastRungIn = false;
end
if isempty(lastRungOut)
    lastRungOut = false;
end
if isempty(lastData)
    lastData = data;
end
if isempty(isInit)
    isInit = true;
else
    isInit = false;
end
if isempty(lastAnimation)
    lastAnimation = false;
end
if isempty(lastDataShow)
    lastDataShow = false;
end

[animation, dataShow] = slplc.utils.setBlockAppearance('set', '%<PLCOperandTag>', {}, {}, ...
    ' = ', {'ForegroundColor'}, ...
    isInit,  ...
    BlockEnable, lastBlockEnable, ...
    RungIn,  lastRungIn, ...
    RungOut, lastRungOut, ...
    data, lastData, ...
    lastAnimation, lastDataShow);

lastBlockEnable = BlockEnable;
lastRungIn      = RungIn;
lastRungOut     = RungOut;
lastData        = data;
lastAnimation   = animation;
lastDataShow    = dataShow;
end

== matlab function fukt_test/PLC Controller Suite/__Logic/Fukt sampling/Fuktmätare sampling/__Logic/MOV/__Format ==
  data: BlockEnable input; RungIn input; RungOut input
function setBlockFormat(BlockEnable, RungIn, RungOut)
% set parent block colors
coder.extrinsic('slplc.utils.setBlockAppearance');
persistent lastBlockEnable lastRungIn lastRungOut isInit lastAnimation lastDataShow;
if isempty(lastBlockEnable)
    lastBlockEnable = true;
end
if isempty(lastRungIn)
    lastRungIn = false;
end
if isempty(lastRungOut)
    lastRungOut = false;
end

if isempty(isInit)
    isInit = true;
else
    isInit = false;
end
if isempty(lastAnimation)
    lastAnimation = false;
end
if isempty(lastDataShow)
    lastDataShow = false;
end

[animation, dataShow] = slplc.utils.setBlockAppearance('set', '', {}, {}, ...
    ' = ',  {'ForegroundColor'}, ...
    isInit,  ...
    BlockEnable, lastBlockEnable, ...
    RungIn,  lastRungIn, ...
    RungOut, lastRungOut, ...
    [],    [], ...
    lastAnimation, lastDataShow);

lastBlockEnable = BlockEnable;
lastRungIn      = RungIn;
lastRungOut     = RungOut;
lastAnimation   = animation;
lastDataShow    = dataShow;
end

== matlab function fukt_test/PLC Controller Suite/__Logic/Fukt sampling/Fuktmätare sampling/__Logic/XIC1/__Format ==
  data: BlockEnable input; RungIn input; RungOut input; data input
function setBlockFormat(BlockEnable, RungIn, RungOut, data)

if data~=0 && data~=1
    error('slplc:inivalidBooleanValue', 'Invalid boolean value %d', data);
end
data = logical(data);

% set parent block colors
coder.extrinsic('slplc.utils.setBlockAppearance');
persistent lastBlockEnable lastRungIn lastRungOut lastData isInit lastAnimation lastDataShow;
if isempty(lastBlockEnable)
    lastBlockEnable = true;
end
if isempty(lastRungIn)
    lastRungIn = false;
end
if isempty(lastRungOut)
    lastRungOut = false;
end
if isempty(lastData)
    lastData = data;
end
if isempty(isInit)
    isInit = true;
else
    isInit = false;
end
if isempty(lastAnimation)
    lastAnimation = false;
end
if isempty(lastDataShow)
    lastDataShow = false;
end

[animation, dataShow] = slplc.utils.setBlockAppearance('set', '%<PLCOperandTag>', {}, {}, ...
    ' = ', {'ForegroundColor'}, ...
    isInit,  ...
    BlockEnable, lastBlockEnable, ...
    RungIn,  lastRungIn, ...
    RungOut, lastRungOut, ...
    data, lastData, ...
    lastAnimation, lastDataShow);

lastBlockEnable = BlockEnable;
lastRungIn      = RungIn;
lastRungOut     = RungOut;
lastData        = data;
lastAnimation   = animation;
lastDataShow    = dataShow;
end

== matlab function fukt_test/PLC Controller Suite/__Logic/Fukt sampling/Fuktmätare sampling/__Logic/RES/Instruction_Enable/Rung-condition-in is true/reset_function ==
  data: y input Bus: TIMER; y output
function y = reset_TIMER(y)

	y.ACC = int32(0);
	y.EN = false;
	y.TT = false;
	y.DN = false;

end

== matlab function fukt_test/PLC Controller Suite/__Logic/Fukt sampling/Fuktmätare sampling/__Logic/XIC2/__Format ==
  data: BlockEnable input; RungIn input; RungOut input; data input
function setBlockFormat(BlockEnable, RungIn, RungOut, data)

if data~=0 && data~=1
    error('slplc:inivalidBooleanValue', 'Invalid boolean value %d', data);
end
data = logical(data);

% set parent block colors
coder.extrinsic('slplc.utils.setBlockAppearance');
persistent lastBlockEnable lastRungIn lastRungOut lastData isInit lastAnimation lastDataShow;
if isempty(lastBlockEnable)
    lastBlockEnable = true;
end
if isempty(lastRungIn)
    lastRungIn = false;
end
if isempty(lastRungOut)
    lastRungOut = false;
end
if isempty(lastData)
    lastData = data;
end
if isempty(isInit)
    isInit = true;
else
    isInit = false;
end
if isempty(lastAnimation)
    lastAnimation = false;
end
if isempty(lastDataShow)
    lastDataShow = false;
end

[animation, dataShow] = slplc.utils.setBlockAppearance('set', '%<PLCOperandTag>', {}, {}, ...
    ' = ', {'ForegroundColor'}, ...
    isInit,  ...
    BlockEnable, lastBlockEnable, ...
    RungIn,  lastRungIn, ...
    RungOut, lastRungOut, ...
    data, lastData, ...
    lastAnimation, lastDataShow);

lastBlockEnable = BlockEnable;
lastRungIn      = RungIn;
lastRungOut     = RungOut;
lastData        = data;
lastAnimation   = animation;
lastDataShow    = dataShow;
end

== matlab function fukt_test/PLC Controller Suite/__Logic/Fukt sampling/Fuktmätare sampling/__Logic/TON1/Instruction_Enable/__Logic ==
  data: EN output; TT output; RungIn input; PRE input; EN input; DN input; DN output; ACC output; ACC input; currentTime input; lastTime input
function [EN, TT, DN, ACC]  = TON(RungIn, PRE, EN, DN, ACC, currentTime, lastTime)
% TON algorithm

if RungIn
    % Rung-condition-in is True
    if PRE < 0 || ACC < 0
        error('slplc:TONError', '.PRE or .ACC cannot be negtive values');
    end
    TT = true;
    if ~DN
        if EN
            deltaT = currentTime - lastTime;
            ACC = ACC + cast(deltaT, class(ACC));
            if ACC == intmax(class(ACC)) || ACC >= PRE
                TT = false;
                DN = true;
            end
        end
    else
        TT = false;
    end
    EN = true;
    % True end
else
    % Rung-condition-in is False
    EN    = false;
    TT    = false;
    DN    = false;
    ACC   = cast(0, class(ACC));
    % False end
end

end

== matlab function fukt_test/PLC Controller Suite/__Logic/Fukt sampling/Fuktmätare sampling/__Logic/TON1/__Format ==
  data: BlockEnable input; RungIn input; RungOut input; data input
function setBlockFormat(BlockEnable, RungIn, RungOut, data)
% set parent block colors
coder.extrinsic('slplc.utils.setBlockAppearance');
persistent lastBlockEnable lastRungIn lastRungOut lastData isInit lastAnimation lastDataShow;
if isempty(lastBlockEnable)
    lastBlockEnable = true;
end
if isempty(lastRungIn)
    lastRungIn = false;
end
if isempty(lastRungOut)
    lastRungOut = false;
end
if isempty(lastData)
    lastData = data;
end
if isempty(isInit)
    isInit = true;
else
    isInit = false;
end
if isempty(lastAnimation)
    lastAnimation = false;
end
if isempty(lastDataShow)
    lastDataShow = false;
end

[animation, dataShow] = slplc.utils.setBlockAppearance('set', '%<PLCBlockType>: %<PLCOperandTag>', {}, {}, ...
    ' = ', {'ForegroundColor'}, ...
    isInit,  ...
    BlockEnable, lastBlockEnable, ...
    RungIn,  lastRungIn, ...
    RungOut, lastRungOut, ...
    data, lastData, ...
    lastAnimation, lastDataShow);

lastBlockEnable = BlockEnable;
lastRungIn      = RungIn;
lastRungOut     = RungOut;
lastData        = data;
lastAnimation   = animation;
lastDataShow    = dataShow;
end

== matlab function fukt_test/PLC Controller Suite/__Logic/Fukt logic/Program/__Logic/OTL1/__Format ==
  data: BlockEnable input; RungIn input; RungOut input; data input
function setBlockFormat(BlockEnable, RungIn, RungOut, data)

if data~=0 && data~=1
    error('slplc:inivalidBooleanValue', 'Invalid boolean value %d', data);
end
data = logical(data);

% set parent block colors
coder.extrinsic('slplc.utils.setBlockAppearance');
persistent lastBlockEnable lastRungIn lastRungOut lastData isInit lastAnimation lastDataShow;
if isempty(lastBlockEnable)
    lastBlockEnable = true;
end
if isempty(lastRungIn)
    lastRungIn = false;
end
if isempty(lastRungOut)
    lastRungOut = false;
end
if isempty(lastData)
    lastData = data;
end
if isempty(isInit)
    isInit = true;
else
    isInit = false;
end
if isempty(lastAnimation)
    lastAnimation = false;
end
if isempty(lastDataShow)
    lastDataShow = false;
end

[animation, dataShow] = slplc.utils.setBlockAppearance('set', '%<PLCOperandTag>', {}, {}, ...
    ' = ', {'ForegroundColor'}, ...
    isInit,  ...
    BlockEnable, lastBlockEnable, ...
    RungIn,  lastRungIn, ...
    RungOut, lastRungOut, ...
    data, lastData, ...
    lastAnimation, lastDataShow);

lastBlockEnable = BlockEnable;
lastRungIn      = RungIn;
lastRungOut     = RungOut;
lastData        = data;
lastAnimation   = animation;
lastDataShow    = dataShow;
end
